simulink model "TD2_Ex1_1_linear"  (R2022a)
settings: Solver=VariableStepAuto  StartTime=0.0  StopTime=20  RelTol=1e-3
undefined symbols (not defined in the file): A, B, eps1, eps2
settings Model: Creator=CS  LastModifiedBy=CS

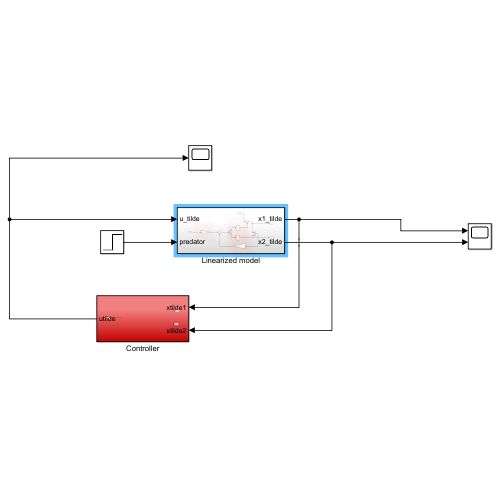
[thumbnail: Simulink's stored preview of the top-level diagram]
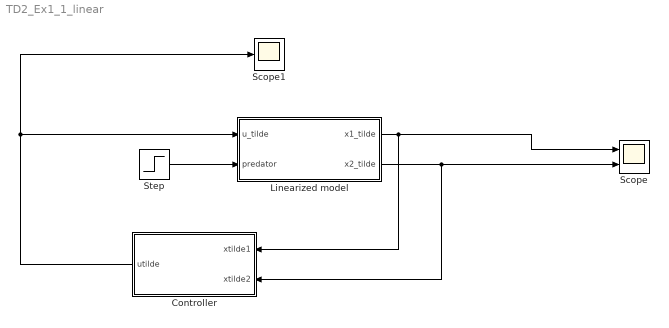
== system TD2_Ex1_1_linear ==
  Controller : Subsystem
  Linearized model : Subsystem
  Scope : Scope  NumInputPorts=2
  Scope1 : Scope
  Step : Step  Time=5  After=0  SampleTime=0
  wires:
  Linearized model/1(x1_tilde) -> Controller/1(xtilde1), Scope/1
  Linearized model/2(x2_tilde) -> Controller/2(xtilde2), Scope/2
  Step/1 -> Linearized model/2(predator)
  Controller/1(utilde) -> Linearized model/1(u_tilde), Scope1/1

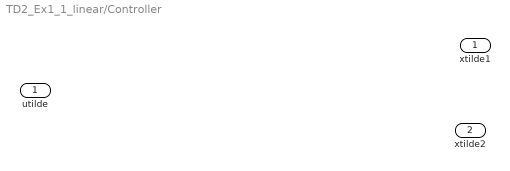
== system TD2_Ex1_1_linear/Controller ==
  xtilde1 : Inport
  xtilde2 : Inport  Port=2
  utilde : Outport
  wires:
  ? -> utilde/1

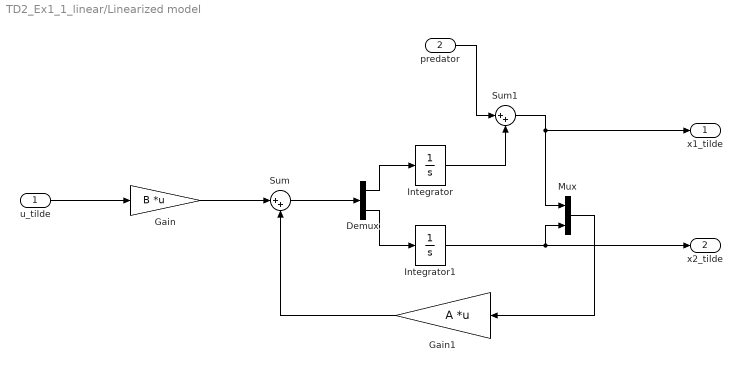
== system TD2_Ex1_1_linear/Linearized model ==
  u_tilde : Inport
  predator : Inport  Port=2
  Demux : Demux  Outputs=2
  Gain : Gain  Gain=B  Multiplication=Matrix(K*u) (u vector)
  Gain1 : Gain  Gain=A  Multiplication=Matrix(K*u) (u vector)
  Integrator : Integrator  InitialCondition=eps1
  Integrator1 : Integrator  InitialCondition=eps2
  Mux : Mux  Inputs=2
  Sum : Sum  Inputs=|++
  Sum1 : Sum  Inputs=|++
  x1_tilde : Outport
  x2_tilde : Outport  Port=2
  wires:
  Demux/2 -> Integrator1/1
  Gain1/1 -> Sum/2
  Integrator1/1 -> Mux/2, x2_tilde/1
  Demux/1 -> Integrator/1
  Sum/1 -> Demux/1
  Mux/1 -> Gain1/1
  Gain/1 -> Sum/1
  u_tilde/1 -> Gain/1
  Integrator/1 -> Sum1/2
  Sum1/1 -> Mux/1, x1_tilde/1
  predator/1 -> Sum1/1
